simulink library "GOcontroll_Moduline_Target"  (R2023b)
settings: Solver=ode45  StartTime=0.0  StopTime=10.0  RelTol=1e-3  EnableMultiTasking=on
PreLoadFcn:
  | compile_gocontroll_mex;
libraries: $bdroot x8, canmsglib x4, simulink x2
(part 1 of 4)
settings Model: Creator=HANcoder  LastModifiedBy=maud
settings Model: ModifiedHistory=|
  | la_obwlf -- Thu Sep 01 12:12:55 2016 -- Version 0.33
  | 
  | 
  | 
  | 
  | 
  | 
  | la_obwlf -- Thu Sep 01 09:23:34 2016 -- Version 0.33
  | changed the version in the Base Sample Time block
  | 
  | 
  | 
  | la_obwlf -- Tue Aug 30 15:48:17 2016 -- Version 0.33
settings SolverCC: AlgebraicLoopSolver=TrustRegion
settings DataIOCC: LimitDataPoints=on  SaveFormat=Array  SignalLoggingSaveFormat=ModelDataLogs  ReturnWorkspaceOutputs=off
settings OptimizationCC: ExpressionDepthLimit=2147483647  LifeSpan=inf
settings DebuggingCC: UnderspecifiedInitializationDetection=Classic  MergeDetectMultiDrivingBlocksExec=none  SolverPrmCheckMsg=warning  FcnCallInpInsideContextMsg=warning  UnconnectedInputMsg=warning  UnconnectedOutputMsg=warning  UnconnectedLineMsg=warning  StateNameClashWarn=warning  SFUnexpectedBacktrackingDiag=warning  SFNoUnconditionalDefaultTransitionDiag=warning  SFExecutionAtInitializationDiag=none  ArithmeticOperatorsInVariantConditions=warning
settings HardwareCC: ProdBitPerPointer=32  ProdBitPerSizeT=32  ProdBitPerPtrDiffT=32  ProdLargestAtomicFloat=None  ProdIntDivRoundTo=Undefined  ProdEndianess=Unspecified  ProdWordSize=32  ProdHWDeviceType=32-bit Generic
settings ModelReferenceCC: EnableRefExpFcnMdlSchedulingChecks=on  PropagateSignalLabelsOutOfModel=off
settings SFSimCC: SimUseLocalCustomCode=off  CustomCodeUndefinedFunction=UseInterfaceOnly
settings RTWCC: RTWUseLocalCustomCode=off
settings CodeAppCC: StateflowObjectComments=on
settings GRTTargetCC: TargetLangStandard=C89/C90 (ANSI)  CombineOutputUpdateFcns=off  GRTInterface=on
settings ConfigComp: CovMetricSettings=dw  CovSaveCumulativeToWorkspaceVar=on  CovSaveSingleToWorkspaceVar=on  CovExternalEMLEnable=off  CovSFcnEnable=off

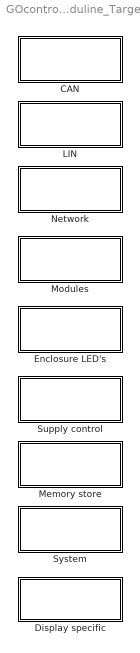
== system GOcontroll_Moduline_Target ==
  CAN : Subsystem
      mask Display: fprintf('CAN');
  Display specific : Subsystem
      mask Display: fprintf("Display specific");
  Enclosure LED's : Subsystem
      mask Display: fprintf('Enclosure LED');
  LIN : Subsystem
      mask Display: fprintf('LIN');
  Memory store : Subsystem
      mask Display: fprintf('Memory store');
  Modules : Subsystem
      mask Display: fprintf('Modules');
  Network : Subsystem
      mask Display: fprintf('Network');
  Supply control : Subsystem
      mask Display: fprintf('Supply Control');
  System : Subsystem
      mask Display: fprintf('System');

== system GOcontroll_Moduline_Target/CAN ==
  " CAN Example" : Subsystem
  CAN 2.0B : Subsystem
      mask Display: fprintf('CAN 2.0B');

== system GOcontroll_Moduline_Target/Display specific ==
  Set display brightness : M-S-Function  FunctionName=sfcn_set_brightness_display  Parameters=tsamp  mask(Set display brightness){tsamp=1}
      mask prompts: tsamp "Sample time:"
      mask help:
      | Set the brightness of a display (only works with the max25014 driver currently)
      | Keeps the original brightness untill the first non zero value is received
      mask Display:
      | fprintf("Set display brightness");
      | text(2, 6, ert_linux_target_version());

== system GOcontroll_Moduline_Target/Enclosure LED's ==
  Enclosure LED : M-S-Function  FunctionName=sfcn_gocontroll_status_led  Parameters=tsamp  mask(Enclosure LED's){tsamp=-1, led=1, color=Red}
      mask prompts: tsamp "Sample time"
      mask help:
      | The Moduline controller is equipped with 4 RGB status LED's. To control them, simply configure the mask ( LED and color) and control them using uint8 values.
      |
      | Note: Moduline IV HW >= 3.02 has duty cycle controlled LED's. The intensity can be set from 0 (0%) to 255 (100%).
      |
      | LED: Select the LED that is needs to be controlled.
      |
      | Color: Select the color the LED needs to illuminate.
      mask init:
      | colorInfoString = {'Red', 'Green', 'Blue'};
      |     colorInfoStr = colorInfoString{color};
      | 
      |     % update RTWdata to run WriteRTW again
      |     modelRTWFields = struct('led', int2str(led),'color', int2str(color));
      |     % Insert modelRTWFields in the I/O block S-Function containing the Tag starting with 'HANcoder_TARGET_'
      |     HANcoder_TARGET_DataBlock = find_system(gcb, 'RegExp', 'on', 'FollowLinks', 'on', 'LookUnderMasks', 'all', 'BlockType', 'M-S-Function');
      |     set_param(HANcoder_TARGET_DataBlock{1}, 'RTWdata', modelRTWFields);
      mask TypeOptions led: 1 | 2 | 3 | 4
      mask TypeOptions color: Red | Green | Blue
      mask Display:
      | fprintf('Status LED %d\nColor: %s',led,colorInfoStr);
      | text(2, 6, ert_linux_target_version());

== system GOcontroll_Moduline_Target/LIN ==
  LIN Master : M-S-Function  FunctionName=sfcn_lin_master  Parameters=tsamp, direction, dataLength  mask(LIN Master){id=0x01, direction=Send data, dataLength=2, check=Classic (LIN 1.3), tsamp=-1}
      mask prompts: id "Identifier"; dataLength "Data Length"; check "Checksum"; tsamp "Sample time"
      mask help:
      | Function
      | ==========
      | This block implements the LIN master functionality for communication with LIN
      | slaves. The block complies with LIN 1.3 an LIN 2.0. When sending data to a slave
      | device, this block will add the data to the LIN bus. When retrieving data from slaves, The block will wait for incoming data over LIN.
      |
      | Parameters
      | ==========
      | Identifier:
      | Selects the identifier to communicate with
      |
      | Direction:
      | Request data from a slave device or send data to a slave device
      |
      | Datalength:
      | Defines the number of bytes that need to be send to- or requested from the slave
      |
      | Checksum:
      | Select Classic for checksum based on databytes only. Enhanced for databytes and
      | ID byte
      |
      | Sample time:
      | Defines the execution interval of the block.
      |
      | Input
      | ==========
      | Port 1..8               LIN Data bytes to be send to a slave
      |
      | Output
      | ==========
      | Port 1..8               LIN Data bytes that are received from the slave
      mask init:
      | % Create resource keywords to be reserved in resource database
      | modelRTWFields = struct('id', int2str(id), 'direction', int2str(direction),'dataLength', int2str(dataLength),'check', int2str(check));
      | 
      | % Insert modelRTWFields in the I/O block S-Function containing the Tag starting with 'HANcoder_TARGET_'
      | HANcoder_TARGET_DataBlock = find_system(gcb, 'RegExp', 'on', 'FollowLinks', 'on', 'LookUnderMasks', 'all', 'BlockType', 'M-S-Function');
      | set_param(HANcoder_TARGET_DataBlock{1}, 'RTWdata', modelRTWFields);
      mask TypeOptions id: 0x01 | 0x02 | 0x03 | 0x04 | 0x05 | 0x06 | 0x07 | 0x08 | 0x09 | 0x0A | 0x0B | 0x0C | 0x0D | 0x0E | 0x0F | 0x10 | 0x11 | 0x12 | 0x13 | 0x14 | 0x15 | 0x16 | 0x17 | 0x18 | 0x19 | 0x1A | 0x1B | 0x1C | 0x1D | 0x1E | 0x1F | 0x20 | 0x21 | 0x22 | 0x23 | 0x24 | 0x25 | 0x26 | 0x27 | 0x28 | 0x29 | 0x2A | 0x2B | 0x2C | 0x2D | 0x2E | 0x2F | 0x30 | 0x31 | 0x32 | 0x33 | 0x34 | 0x35 | 0x36 | 0x37 | 0x38 | 0x39 | 0x3A | 0x3B | 0x3C (diagnostic) | 0x3D (diagnostic) | 0x3E (reserved) | 0x3F (reserved)
      mask TypeOptions direction: Request data | Send data
      mask TypeOptions dataLength: 2 | 4 | 8
      mask TypeOptions check: Classic (LIN 1.3) | Enhanced (LIN 2.0)
      mask Display:
      | fprintf('Master LIN\nmessage\nID: 0x%x',id);
      | text(2, 6, ert_linux_target_version());
      | if direction == 1
      |     port_label('output', 1, 'byte 1');
      |     port_label('output', 2, 'byte 2');
      |     if dataLength > 1
      |         port_label('output', 3, 'byte 3');
      |         port_label('output', 4, 'byte 4');
      |     end
      |     if dataLength > 2
      |         port_label('output', 5, 'byte 5');
      |         port_label('output', 6, 'byte 6');
      |         port_label('output', 7, 'byte 7');
      |         port_label('output', 8, 'byte 8');
      |     end
      | else
      |     port_label('input', 1, 'byte 1');
      |     port_label('input', 2, 'byte 2');
      |     if dataLength > 1
      |         port_label('input', 3, 'byte 3');
      |         port_label('input', 4, 'byte 4');
      |     end
      |     if dataLength > 2
      |         port_label('input', 5, 'byte 5');
      |         port_label('input', 6, 'byte 6');
      |         port_label('input', 7, 'byte 7');
      |         port_label('input', 8, 'byte 8');
      |     end
      | end

== system GOcontroll_Moduline_Target/Memory store ==
  Diagnostic to memory : Subsystem
      mask Display: fprintf('Diagnostic to memory');
  Variable to memory : Subsystem
      mask Display: fprintf('Variable to memory');

== system GOcontroll_Moduline_Target/Modules ==
  Bridge Module : Subsystem
      mask Display: fprintf('Bridge Module');
  Input Module : Subsystem
      mask Display: fprintf('Input Module');
  Output Module : Subsystem
      mask Display: fprintf('Output Module');

== system GOcontroll_Moduline_Target/Network ==
  MQTT : Subsystem  Commented=on
      mask Display: fprintf('MQTT');
  TCP : Subsystem
      mask Display: fprintf('TCP');
  UDP : Subsystem
      mask Display: fprintf('UDP');

== system GOcontroll_Moduline_Target/Supply control ==
  Controller Active : M-S-Function  FunctionName=sfcn_gocontroll_controller_active  Parameters=tsamp  mask(Controller Active){tsamp=1}
      mask prompts: tsamp "Sample time"
      mask help:
      | The GOcontroll Moduline IV is able to keep itself alive. As long the K30 power is applied (connector C pin 5-7) and the input of the Controller Active function block is high, the controller will stay on even if the K15 pins (connector C pin 2,3 or 4) are low.
      | If the controller is switched off by software, a restart is only possible when the device is activated by one of the K15 pins of connector C.
      |
      | To detect an external shutdown (K15 pins goes low), simply drag in the K15 Voltage block. This block provides the input voltage from the K15 pins
      mask Display:
      | fprintf('Controller Active');
      | text(2, 6, ert_linux_target_version());
  K15 Voltage : M-S-Function  FunctionName=sfcn_gocontroll_k15_voltage  Parameters=tsamp,k15pin  mask(Contact Voltage){ContrType=GOcontroll Moduline IV, tsamp=1, k15pin=K15-1 (Connector C pin 2)}
      mask prompts: ContrType "Controller Type"; tsamp "Sample time"; k15pin "K15 input pin"
      mask help: The K15 voltage provides the K15 voltage in mV that is applied on the K15 pins of the controller. A positive voltage on one of these pins will start-up the controller. These function blocks can be used to read out which K15 input pin triggered the startup.
      mask init:
      | %update RTWdata to run WriteRTW again
      |     modelRTWFields = struct('k15pin', int2str(k15pin));
      |     % Insert modelRTWFields in the I/O block S-Function containing the Tag starting with 'HANcoder_TARGET_'
      |     HANcoder_TARGET_DataBlock = find_system(gcb, 'RegExp', 'on', 'FollowLinks', 'on', 'LookUnderMasks', 'all', 'BlockType', 'M-S-Function');
      |     set_param(HANcoder_TARGET_DataBlock{1}, 'RTWdata', modelRTWFields);
      mask TypeOptions ContrType: GOcontroll Moduline IV | GOcontroll Moduline Mini | GOcontroll Moduline Display
      mask Callback ContrType:
      | controller = get_param(gcb, 'ContrType');
      | mask = Simulink.Mask.get(gcb);
      | adc = mask.getParameter('k15pin');
      | 
      | if(controller == "GOcontroll Moduline IV")
      |     adc.TypeOptions = {'K15-1 (Connector C pin 2)','K15-2 (Connector C pin 3)','K15-3 (Connector C pin 4)'};
      | elseif (controller == "GOcontroll Moduline Mini")
      |     adc.TypeOptions = {'K15-1 (Connector B pin 17)','K15-2 (Connector A pin 16)','K15-3 (Connector A pin 17)'};
      | elseif (controller == "GOcontroll Moduline Display")
      |     adc.TypeOptions = {'K15 (Connector A pin 9)','Sensor (6 pin Minitek pin 3)','Adapter board Sensor'};
      | end
      mask TypeOptions k15pin: K15-1 (Connector C pin 2) | K15-2 (Connector C pin 3) | K15-3 (Connector C pin 4)
      mask Display:
      | fprintf('ADC voltage\n%s',get_param(gcb, 'k15pin'));
      | text(2, 6, ert_linux_target_version());
  K30 Voltage : M-S-Function  FunctionName=sfcn_gocontroll_k30_voltage  Parameters=tsamp  mask(Supply voltage){ContrType=GOcontroll Moduline IV, tsamp=1}
      mask prompts: ContrType "Controller type"; tsamp "Sample time"
      mask help: The K30 voltage provides the power supply in mV that is applied on the K30 pins.
      mask TypeOptions ContrType: GOcontroll Moduline IV | GOcontroll Moduline Mini | GOcontroll Moduline Display
      mask Display:
      | if ContrType == 1
      |     fprintf('K30 Voltage\nConnector C pin 5-7');
      | elseif ContrType == 2
      |     fprintf('K30 Voltage\nConnector B pin 8-9');
      | elseif ContrType == 3
      |     fprintf('K30 Voltage\nConnector A pin 9');
      | end
      | text(2, 6, ert_linux_target_version());

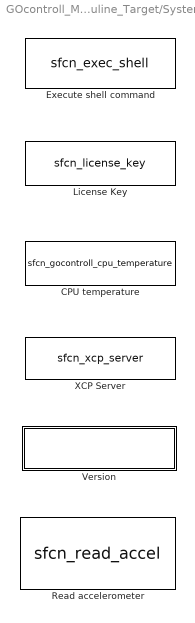
== system GOcontroll_Moduline_Target/System ==
  CPU temperature : M-S-Function  FunctionName=sfcn_gocontroll_cpu_temperature  Parameters=tsamp  mask(Get CPU temperature){tsamp=1}
      mask prompts: tsamp "Sample time"
      mask help: Block to retrieve the CPU temperature of the i.MX core
      mask Display:
      | fprintf('Get CPU temperature');
      | text(2, 6, ert_linux_target_version());
  Execute shell command : M-S-Function  FunctionName=sfcn_exec_shell  mask(Execute shell command){command='command'}
      mask help:
      | Execute a Linux Shell command when the input is true.
      |
      | Accepts a Boolean input, use a triggered subsystem to call the function only once on a state change instead of every sample.
      mask init:
      | if ~ischar(command)
      |         error('Given command is not a string');
      |     end
      | 
      |     %update RTWdata so WriteRTW gets called again
      |     modelRTWFields = struct('command', command);
      | 
      |     % Insert modelRTWFields in the I/O block S-Function containing the Tag starting with 'HANcoder_TARGET_'
      |     HANcoder_TARGET_DataBlock = find_system(gcb, 'RegExp', 'on', 'FollowLinks', 'on', 'LookUnderMasks', 'all', 'BlockType', 'M-S-Function');
      |     set_param(HANcoder_TARGET_DataBlock{1}, 'RTWdata', modelRTWFields);
      mask Display:
      | fprintf("Execute command:\n%s",command);
      | text(2, 6, ert_linux_target_version());
  License Key : M-S-Function  FunctionName=sfcn_license_key  Parameters=key,iv,license,check_file  mask(Check software license key){key=[1 2 3 4 5 6 7 8 9 10 11 12 13 14 15 16], iv='init vec', license='path/to/license', check_file='path/to/checkfile'}
      mask prompts: key "Encryption key"; iv "Initialisation vector"; license "License file"; check_file "Check file"
      mask help:
      | Function block to check the controller for a license key upon executing the software.
      |
      | example lines are literal to what should be in the field
      |
      | Encryption key:
      |
      | An array of 16, 24 or 32 bytes, for example:
      | hex2dec(["0x01", "0x23", "0x45", "0x67", "0x89", "0xAB", "0xCD", "0xEF", "0x01", "0x23", "0x45", "0x67", "0x89", "0xAB", "0xCD", "0xEF"])
      |
      | bytes can be written in any form accepted by the c compiler: 0x00/0 to 0xFf/255.
      |
      | Inititialisation vector:
      |
      | A string of characters (max 16 bytes) example:
      | '123kdgh34ndfg84'
      |
      |
      | License file:
      |
      | A string containing the path to the license file, example:
      | '/etc/simulink/license'
      |
      |
      | Check file:
      |
      | A string containing the path to the license file, example:
      | '/etc/simulink/check_file'
      |
      |
      | Method of operation:
      | This block uses the <a href="https://github.com/jhjin/OpenAES">OpenAES library</a>. It also has a tool that can be used to generate an encryption key and to encrypt a file with said key.
      |
      | This block will attempt to decrypt the "license file" with the given key and initialisation vector, it will then be compared to the "check file". If these match the program is allowed to continue.
      |
      | To make this work effectively it is essential to encrypt a file that is unique for the system and can't be easily edited. for example "/sys/class/net/eth0/address".
      |
      | An important note with using this block is that the bytes of the key are swapped and so need to be entered slightly differently in this block, for example:
      | key: byte 1 byte 2 byte 3 byte 4 byte 5 byte 6 ...
      | block: {byte 2, byte 1, byte 4, byte 3, byte 6, byte 5, ...}
      |
      | If the model terminates with the error:
      | Error: Failed to decrypt2. return code: ##
      mask init:
      | if ~(length(key) == 16 || length(key) == 24 || length(key) == 32)
      |         error('Encrypion key has an invalid length, it should be 16, 24 or 32 bytes long');
      |     end
      |     for idx = 1:length(key)
      |         if key(idx) > 255 || key(idx) < 0 || mod(key(idx),1) > 0
      |             error('Encryption key does not consist of values that match a uint8');
      |         end
      |     end
      |     if ~ischar(iv)
      |         error('Initialisation vector should be a string');
      |     end
      |     if ~ischar(license)
      |         error('Path to the license file should be a string');
      |     end
      |     if ~ischar(check_file)
      |         error('Path to the check file should be a string');
      |     end
      | 
      |     %update RTWdata here so the WriteRTW callback gets run again
      |     modelRTWFields = struct('key', mat2str(key), 'iv', iv, 'license', license, 'check_file', check_file, 'key_len', num2str(length(key)));
      | 
      |     set_param(gcb, 'RTWdata', modelRTWFields);
      mask Display:
      | fprintf('Check software license');
      | text(2, 6, ert_linux_target_version());
  Read accelerometer : M-S-Function  FunctionName=sfcn_read_accel  Parameters=tsamp  mask(Read accelerometer){sampling_frequency=12, scale=-2G/2G, tsamp=0.1}
      mask prompts: sampling_frequency "Chip sampling frequency in Hz"; scale "Sensitivity"; tsamp "Sample time"
      mask help:
      | This block reads out the accelerometer that is present on the moduline mini, other controllers will not work with this block.
      |
      | It outputs the acceleration in all 3 spatial dimensons in m/s^2.
      |
      | Positive X axis is acceleration towards the connectors in the length of the controller
      | Positive Y axis is acceleration towards the empty side of the controller, so opposite of the two m12 connectors
      | Positive Z axis is acceleration straight up if the controller was lying on its back so towards the indicator leds
      mask init:
      | switch get_param(gcb, 'scale')
      |     case '-2G/2G'
      |         scale_factor = '0.009571';
      |     case '-4G/4G'
      |         scale_factor = '0.019142';
      |     case '-8G/8G'
      |         scale_factor = '0.038285';
      |     case '-16G/16G'
      |         scale_factor = '0.076570';
      |     otherwise
      |         error('invalid sensitivity selected');
      | end
      | 
      | modelRTWFields = struct('sampling_frequency', get_param(gcb, 'sampling_frequency'), 'scale', scale_factor);
      | 
      | set_param(gcb, 'RTWdata', modelRTWFields);
      mask TypeOptions sampling_frequency: 1 | 12 | 25 | 50 | 100 | 200
      mask TypeOptions scale: -2G/2G | -4G/4G | -8G/8G | -16G/16G
      mask Display:
      | fprintf('Read accelerometer\nChip sampling frequency: %s Hz', get_param(gcb,'sampling_frequency'));
      | 
      | port_label('output', 1, 'X');
      | port_label('output', 2, 'Y');
      | port_label('output', 3, 'Z');
      | 
      | text(2, 6, ert_linux_target_version());
  Version : Subsystem  mask{major=0, feature=0, fix=1}
      mask help:
      | This block helps with keeping track of the model version.
      |
      | The values entered will be written to /usr/mem-sim/[MODEL_MAJOR,MODEL_FEATURE,MODEL_FIX].
      |
      | They are also available to use in the model with a From block, consider making them ExportedGlobal this way.
      mask init:
      | if mod(major,1) > 0
      |         error("Major must be an integer value");
      |     end
      |     if mod(feature,1) > 0
      |         error("Feature must be an integer value");
      |     end
      |     if mod(fix,1) > 0
      |         error("Fix must be an integer value");
      |     end
      mask TypeOptions major: Initialize Function/Major/Value
      mask TypeOptions feature: Initialize Function/Feature/Value
      mask TypeOptions fix: Initialize Function/Fix/Value
      mask Display:
      | fprintf('Model V%s.%s.%s', int2str(major), int2str(feature), int2str(fix));
      | text(2, 6, ert_linux_target_version());
  XCP Server : M-S-Function  Priority=999999  FunctionName=sfcn_xcp_server  mask(XCP Server){server_type=TCP}
      mask prompts: server_type "Server type"
      mask help: Having one block of this type in your model enables the XCP server to use with HANtune
      mask init:
      | %update RTWdata here so the WriteRTW callback gets run again
      |     modelRTWFields = struct('server_type', int2str(server_type));
      | 
      |     set_param(gcb, 'RTWdata', modelRTWFields);
      mask TypeOptions server_type: TCP | UDP
      mask Display:
      | fprintf('XCP Server\n%s', get_param(gcb,'server_type'));
      | text(2, 6, ert_linux_target_version());

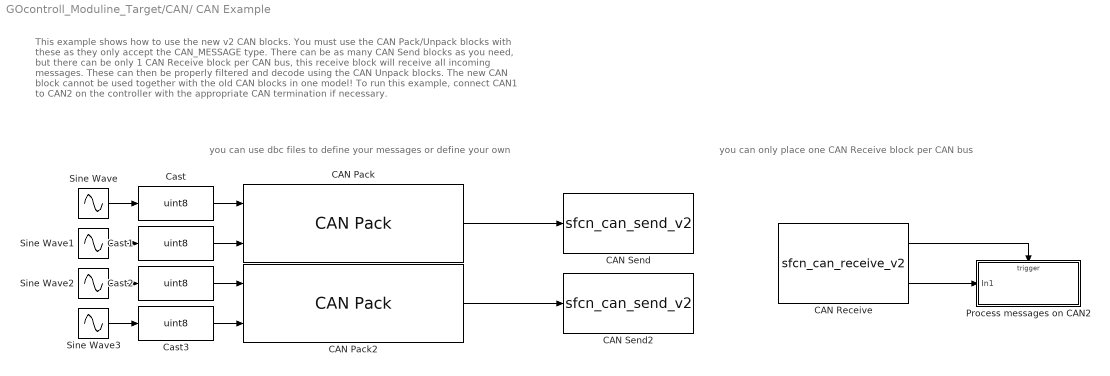
== system GOcontroll_Moduline_Target/CAN/ CAN Example ==
  note: This example shows how to use the new v2 CAN blocks.
      | You must use the CAN Pack/Unpack blocks with these as they only accept the CAN_MESSAGE type.
      | There can be as many CAN Send blocks as you need, but there can be only 1 CAN Receive block per CAN bus, this receive block will receive all incoming messages.
      | These can then be properly filtered and decode using the CAN Unpack blocks.
      | The new CAN block cannot be used together with the old CAN blocks in one model!
      |
      | To run this example, connect CAN1 to CAN2 on the controller with the appropriate CAN termination if necessary.
  note: you can use dbc files to define your messages or define your own
  note: you can only place one CAN Receive block per CAN bus
  CAN Pack : canmsglib/CAN Pack  MsgList=(none)  MsgName=CAN Msg  MsgIDType=Standard (11-bit identifier)  MsgIdentifier=10  MsgLength=2  Remote=off  ApplyMinMax=off  BusOutput=off  SignalInfo={ 'led1', '0', '8', 'LE', 'unsigned', 'Standard', '0', '1', '0', '-Inf', 'Inf'; 'led2', '8', '8', 'LE', 'unsigned', 'Standard', '0', '1', '0', '-Inf', 'Inf' }
      settings: LibrarySourceBlock=embeddedtargetslib/Host Communication/CAN Pack  DataFormat=manually specified signals
  CAN Pack2 : canmsglib/CAN Pack  MsgList=(none)  MsgName=CAN Msg  MsgIDType=Standard (11-bit identifier)  MsgIdentifier=11  MsgLength=2  Remote=off  ApplyMinMax=off  BusOutput=off  SignalInfo={ 'led3', '0', '8', 'LE', 'unsigned', 'Standard', '0', '1', '0', '-Inf', 'Inf'; 'led4', '8', '8', 'LE', 'unsigned', 'Standard', '0', '1', '0', '-Inf', 'Inf' }
      settings: LibrarySourceBlock=embeddedtargetslib/Host Communication/CAN Pack  DataFormat=manually specified signals
  CAN Receive : S-Function  AncestorBlock=GOcontroll_Moduline_Target/CAN/CAN 2.0B/CAN Receive  FunctionName=sfcn_can_receive_v2  Parameters=module_id, tsamp  SFunctionDeploymentMode=off  EnableBusSupport=off  mask(CAN Receive){ContrType=GOcontroll Moduline Mini, module_id=CAN2 - Connector A pin 24 (L) and pin 25 (H), tsamp=-1}
      mask prompts: ContrType "Controller Type"; module_id "CAN Bus"; tsamp "Sample time"
      mask help:
      | <p>Receive a messages from the CAN bus.</p>
      | <p>The output is a CAN_MESSAGE object. CAN Unpack block can be used to unpack the data from CAN_MESSAGE object.</p>
      | <p>A Function-call subsystem is triggered every time when a new message has been received.</p>
      | <p>There can be only one receive block on a given CAN bus, this receive block will receive all CAN messages on this bus. To filter them use the CAN Unpack blocks inside of a function call subsystem</p>
      mask TypeOptions ContrType: GOcontroll Moduline IV | GOcontroll Moduline Mini | GOcontroll Moduline Display
      mask Callback ContrType:
      | controller = get_param(gcb, 'ContrType');
      | mask = Simulink.Mask.get(gcb);
      | can_ifs = mask.getParameter('module_id');
      | 
      | if(controller == "GOcontroll Moduline IV")
      | can_ifs.TypeOptions = {'CAN1 - Connector C pin 14 (L) and pin 15 (H)','CAN2 - Connector C pin 20 (L) and pin 21 (H)',...
      |     'CAN3 - Connector C pin 19 (L) and pin 18 (H)','CAN4 - Connector C pin 13 (L) and pin 12 (H)'};
      | elseif (controller == "GOcontroll Moduline Mini")
      |  can_ifs.TypeOptions = {'CAN1 - Connector B pin 24 (L) and pin 25 (H)','CAN2 - Connector A pin 24 (L) and pin 25 (H)'};
      | 
      | elseif (controller == "GOcontroll Moduline Display")
      | can_ifs.TypeOptions = {'CAN1 - Connector A pin 16 (L) and pin 17 (H)','CAN2 - Connector A pin 24 (L) and pin 25 (H)'};
      | end
      mask TypeOptions module_id: CAN1 - Connector B pin 24 (L) and pin 25 (H) | CAN2 - Connector A pin 24 (L) and pin 25 (H)
      mask Display:
      | fprintf('Receive on\nCAN %x', module_id);
      | 
      | port_label('output', 1, 'function call');
      | port_label('output', 2, 'message');
      | text(2, 6, ert_linux_target_version());
  CAN Send : S-Function  AncestorBlock=GOcontroll_Moduline_Target/CAN/CAN 2.0B/CAN Send  FunctionName=sfcn_can_send_v2  Parameters=module_id, tsamp  SFunctionDeploymentMode=off  EnableBusSupport=off  mask(CAN Send){ContrType=GOcontroll Moduline Mini, module_id=CAN1, tsamp=0.01}
      mask prompts: ContrType "Controller Type"; module_id "Module"; tsamp "Sample time"
      mask help:
      | <p>Send a CAN message.</p>
      | <p>Expects a CAN_MESSAGE object as an input. Use CAN Pack to create the CAN_MESSAGE object.</p>
      mask TypeOptions ContrType: GOcontroll Moduline IV | GOcontroll Moduline Mini | GOcontroll Moduline Display
      mask Callback ContrType:
      | controller = get_param(gcb, 'ContrType');
      | mask = Simulink.Mask.get(gcb);
      | can_ifs = mask.getParameter('module_id');
      | 
      | if(controller == "GOcontroll Moduline IV")
      |     can_ifs.TypeOptions = {'CAN1 - Connector C pin 14 (L) and pin 15 (H)','CAN2 - Connector C pin 20 (L) and pin 21 (H)',...
      |         'CAN3 - Connector C pin 19 (L) and pin 18 (H)','CAN4 - Connector C pin 13 (L) and pin 12 (H)'};
      | elseif (controller == "GOcontroll Moduline Mini")
      |     can_ifs.TypeOptions = {'CAN1 - Connector B pin 24 (L) and pin 25 (H)','CAN2 - Connector A pin 24 (L) and pin 25 (H)'};
      | 
      | elseif (controller == "GOcontroll Moduline Display")
      |     can_ifs.TypeOptions = {'CAN1 - Connector A pin 16 (L) and pin 17 (H)','CAN2 - Connector A pin 24 (L) and pin 25 (H)'};
      | end
      mask TypeOptions module_id: CAN1 - Connector B pin 24 (L) and pin 25 (H) | CAN2 - Connector A pin 24 (L) and pin 25 (H)
      mask Display:
      | fprintf('Send on\nCAN%x', module_id);
      | port_label('input', 1, 'Msg');
      | 
      | text(2, 6, ert_linux_target_version());
  CAN Send2 : S-Function  AncestorBlock=GOcontroll_Moduline_Target/CAN/CAN 2.0B/CAN Send  FunctionName=sfcn_can_send_v2  Parameters=module_id, tsamp  SFunctionDeploymentMode=off  EnableBusSupport=off  mask(CAN Send){ContrType=GOcontroll Moduline Mini, module_id=CAN1, tsamp=0.01}
      mask prompts: ContrType "Controller Type"; module_id "Module"; tsamp "Sample time"
      mask help:
      | <p>Send a CAN message.</p>
      | <p>Expects a CAN_MESSAGE object as an input. Use CAN Pack to create the CAN_MESSAGE object.</p>
      mask TypeOptions ContrType: GOcontroll Moduline IV | GOcontroll Moduline Mini | GOcontroll Moduline Display
      mask Callback ContrType:
      | controller = get_param(gcb, 'ContrType');
      | mask = Simulink.Mask.get(gcb);
      | can_ifs = mask.getParameter('module_id');
      | 
      | if(controller == "GOcontroll Moduline IV")
      |     can_ifs.TypeOptions = {'CAN1 - Connector C pin 14 (L) and pin 15 (H)','CAN2 - Connector C pin 20 (L) and pin 21 (H)',...
      |         'CAN3 - Connector C pin 19 (L) and pin 18 (H)','CAN4 - Connector C pin 13 (L) and pin 12 (H)'};
      | elseif (controller == "GOcontroll Moduline Mini")
      |     can_ifs.TypeOptions = {'CAN1 - Connector B pin 24 (L) and pin 25 (H)','CAN2 - Connector A pin 24 (L) and pin 25 (H)'};
      | 
      | elseif (controller == "GOcontroll Moduline Display")
      |     can_ifs.TypeOptions = {'CAN1 - Connector A pin 16 (L) and pin 17 (H)','CAN2 - Connector A pin 24 (L) and pin 25 (H)'};
      | end
      mask TypeOptions module_id: CAN1 - Connector B pin 24 (L) and pin 25 (H) | CAN2 - Connector A pin 24 (L) and pin 25 (H)
      mask Display:
      | fprintf('Send on\nCAN%x', module_id);
      | port_label('input', 1, 'Msg');
      | 
      | text(2, 6, ert_linux_target_version());
  Cast{,1..3} (4 alike) : DataTypeConversion  OutDataTypeStr=uint8  SaturateOnIntegerOverflow=off  RndMeth=Floor
  Process messages on CAN2 : Subsystem  TreatAsAtomicUnit=on
  Sine Wave{,1..3} (4 alike) : Sin  SineType=Sample based  Amplitude=100  Bias=100  Samples=200  SampleTime=0.01
  wires:
  CAN Pack2/1 -> CAN Send2/1
  CAN Receive/2 -> Process messages on CAN2/1(In1)
  CAN Receive/1 -> Process messages on CAN2/Trigger
  Cast3/1 -> CAN Pack2/2
  Cast2/1 -> CAN Pack2/1
  Cast1/1 -> CAN Pack/2
  Sine Wave3/1 -> Cast3/1
  Sine Wave2/1 -> Cast2/1
  Sine Wave1/1 -> Cast1/1
  Sine Wave/1 -> Cast/1
  Cast/1 -> CAN Pack/1
  CAN Pack/1 -> CAN Send/1

== system GOcontroll_Moduline_Target/CAN/CAN 2.0B ==
  CAN Receive : S-Function  FunctionName=sfcn_can_receive_v2  Parameters=module_id, tsamp  SFunctionDeploymentMode=off  EnableBusSupport=off  mask(CAN Receive){ContrType=GOcontroll Moduline IV, module_id=CAN1, tsamp=-1}
      mask prompts: ContrType "Controller Type"; module_id "CAN Bus"; tsamp "Sample time"
      mask help:
      | <p>Receive a messages from the CAN bus.</p>
      | <p>The output is a CAN_MESSAGE object. CAN Unpack block can be used to unpack the data from CAN_MESSAGE object.</p>
      | <p>A Function-call subsystem is triggered every time when a new message has been received.</p>
      | <p>There can be only one receive block on a given CAN bus, this receive block will receive all CAN messages on this bus. To filter them use the CAN Unpack blocks inside of a function call subsystem</p>
      mask TypeOptions ContrType: GOcontroll Moduline IV | GOcontroll Moduline Mini | GOcontroll Moduline Display
      mask Callback ContrType:
      | controller = get_param(gcb, 'ContrType');
      | mask = Simulink.Mask.get(gcb);
      | can_ifs = mask.getParameter('module_id');
      | 
      | if(controller == "GOcontroll Moduline IV")
      | can_ifs.TypeOptions = {'CAN1 - Connector C pin 14 (L) and pin 15 (H)','CAN2 - Connector C pin 20 (L) and pin 21 (H)',...
      |     'CAN3 - Connector C pin 19 (L) and pin 18 (H)','CAN4 - Connector C pin 13 (L) and pin 12 (H)'};
      | elseif (controller == "GOcontroll Moduline Mini")
      |  can_ifs.TypeOptions = {'CAN1 - Connector B pin 24 (L) and pin 25 (H)','CAN2 - Connector A pin 24 (L) and pin 25 (H)'};
      | 
      | elseif (controller == "GOcontroll Moduline Display")
      | can_ifs.TypeOptions = {'CAN1 - Connector A pin 16 (L) and pin 17 (H)','CAN2 - Connector A pin 24 (L) and pin 25 (H)'};
      | end
      mask TypeOptions module_id: CAN1 - Connector C pin 14 (L) and pin 15 (H) | CAN2 - Connector C pin 20 (L) and pin 21 (H) | CAN3 - Connector C pin 19 (L) and pin 18 (H) | CAN4 - Connector C pin 13 (L) and pin 12 (H)
      mask Display:
      | fprintf('Receive on\nCAN %x', module_id);
      | 
      | port_label('output', 1, 'function call');
      | port_label('output', 2, 'message');
      | text(2, 6, ert_linux_target_version());
  CAN Send : S-Function  FunctionName=sfcn_can_send_v2  Parameters=module_id, tsamp  SFunctionDeploymentMode=off  EnableBusSupport=off  mask(CAN Send){ContrType=GOcontroll Moduline IV, module_id=CAN1, tsamp=0.1}
      mask prompts: ContrType "Controller Type"; module_id "CAN Bus"; tsamp "Sample time"
      mask help:
      | <p>Send a CAN message.</p>
      | <p>Expects a CAN_MESSAGE object as an input. Use CAN Pack to create the CAN_MESSAGE object.</p>
      mask TypeOptions ContrType: GOcontroll Moduline IV | GOcontroll Moduline Mini | GOcontroll Moduline Display
      mask Callback ContrType:
      | controller = get_param(gcb, 'ContrType');
      | mask = Simulink.Mask.get(gcb);
      | can_ifs = mask.getParameter('module_id');
      | 
      | if(controller == "GOcontroll Moduline IV")
      |     can_ifs.TypeOptions = {'CAN1 - Connector C pin 14 (L) and pin 15 (H)','CAN2 - Connector C pin 20 (L) and pin 21 (H)',...
      |         'CAN3 - Connector C pin 19 (L) and pin 18 (H)','CAN4 - Connector C pin 13 (L) and pin 12 (H)'};
      | elseif (controller == "GOcontroll Moduline Mini")
      |     can_ifs.TypeOptions = {'CAN1 - Connector B pin 24 (L) and pin 25 (H)','CAN2 - Connector A pin 24 (L) and pin 25 (H)'};
      | 
      | elseif (controller == "GOcontroll Moduline Display")
      |     can_ifs.TypeOptions = {'CAN1 - Connector A pin 16 (L) and pin 17 (H)','CAN2 - Connector A pin 24 (L) and pin 25 (H)'};
      | end
      mask TypeOptions module_id: CAN1 - Connector C pin 14 (L) and pin 15 (H) | CAN2 - Connector C pin 20 (L) and pin 21 (H) | CAN3 - Connector C pin 19 (L) and pin 18 (H) | CAN4 - Connector C pin 13 (L) and pin 12 (H)
      mask Display:
      | fprintf('Send on\nCAN%x', module_id);
      | port_label('input', 1, 'Msg');
      | 
      | text(2, 6, ert_linux_target_version());
  CAN receive1 : M-S-Function  FunctionName=sfcn_can_receive  Parameters=tsamp,canBus,outputNumber,dataType, byteOrder  mask(CAN receive (Legacy)){ContrType=GOcontroll Moduline IV, canBus=CAN1 - Connector C pin 14 (L) and pin 15 (H), outputNumber=1, dataType=uint8, byteOrder=on, tsamp=-1}
      mask prompts: ContrType "Controller Type"; canBus "CAN channel"; outputNumber "Output ports"; dataType "Output datatype"; byteOrder "Byte order: Checked = MSB first, unchecked = LSB first."; tsamp "Sample time"
      mask help:
      | !! Legacy block, use the CAN receive instead of CAN receive1 in future projects !!
      | !! These will not work together, either use the legacy blocks or the new ones !!
      |
      | Function
      | ==========
      | Receive the newest message from the specified CAN channel.
      |
      | Parameters
      | ==========
      | Controller Type          The controller type, only changes the available CAN channels and puts the correct pinout for that type
      | CAN channel:             The CAN channel to send the message on.
      | Output ports:             The amount of output ports
      | Output datatype:       The datatype of the output ports
      | Byte order:                 Select MSB or LSB first
      | Sample time:              -1 or divisible by base sample time [seconds]
      |
      | Input
      | ==========
      | Port 1:                       CAN ID(uint32) in hexadecimal ie: hex2dec('0a')
      |
      | Output
      | ==========
      | Port 1:                       Checks for new message(int8)
      | Port 2..9                     Message data
      mask init:
      | % calculate the data length (targe specific)
      | dataLength = 0;
      | switch(dataType)
      |     case {1,2,7}
      |         % data length of 1 byte
      |         dataLength = outputNumber * 1;
      |     case {3,4}
      |         % data length of 2 bytes
      |         dataLength = outputNumber * 2;
      |     case {5,6}
      |         % data length of 4 bytes
      |         dataLength = outputNumber * 4;
      | end
      | 
      | % check if number of outputs, combined with the data type, is exceeding the
      | % maximum data length
      | if (dataLength < 1)
      |     error ('The CAN message has a minimum of 1 byte');
      | elseif (dataLength > 8)
      |     error('The CAN message supports only up to 8 data bytes');
      | end
      | 
      | % Create resource keywords to be reserved in resource database
      | modelRTWFields = struct('canBus', int2str(canBus-1),...
      |     'outputNumber', int2str(outputNumber), 'dataType', int2str(dataType), 'byteOrder', int2str(byteOrder),...
      |     'dataLength', int2str(dataLength));
      | 
      | set_param(gcb, 'RTWdata', modelRTWFields);
      mask TypeOptions ContrType: GOcontroll Moduline IV | GOcontroll Moduline Mini | GOcontroll Moduline Display
      mask Callback ContrType:
      | controller = get_param(gcb, 'ContrType');
      | mask = Simulink.Mask.get(gcb);
      | can_ifs = mask.getParameter('canBus');
      | 
      | if(controller == "GOcontroll Moduline IV")
      |     can_ifs.TypeOptions = {'CAN1 - Connector C pin 14 (L) and pin 15 (H)','CAN2 - Connector C pin 20 (L) and pin 21 (H)',...
      |         'CAN3 - Connector C pin 19 (L) and pin 18 (H)','CAN4 - Connector C pin 13 (L) and pin 12 (H)'};
      | elseif (controller == "GOcontroll Moduline Mini")
      |     can_ifs.TypeOptions = {'CAN1 - Connector B pin 24 (L) and pin 25 (H)','CAN2 - Connector A pin 24 (L) and pin 25 (H)'};
      | 
      | elseif (controller == "GOcontroll Moduline Display")
      |     can_ifs.TypeOptions = {'CAN1 - Connector A pin 16 (L) and pin 17 (H)','CAN2 - Connector A pin 24 (L) and pin 25 (H)'};
      | end
      mask TypeOptions canBus: CAN1 - Connector C pin 14 (L) and pin 15 (H) | CAN2 - Connector C pin 20 (L) and pin 21 (H) | CAN3 - Connector C pin 19 (L) and pin 18 (H) | CAN4 - Connector C pin 13 (L) and pin 12 (H)
      mask TypeOptions dataType: int8 | uint8 | int16 | uint16 | int32 | uint32 | boolean
      mask Display:
      | fprintf('Receive on\nCAN %x', canBus);
      | port_label('output', 1, 'new')
      | port_label('input', 1, 'ID');
      | text(2, 6, ert_linux_target_version());
  CAN send1 : M-S-Function  FunctionName=sfcn_can_send  Parameters=tsamp, canBus, frameType, inputNumber,RTR  mask(CAN send (Legacy)){ContrType=GOcontroll Moduline IV, canBus=CAN1 - Connector C pin 14 (L) and pin 15 (H), frameType=Standard (11 bit), inputNumber=1, RTR=off, tsamp=-1}
      mask prompts: ContrType "Controller Type"; canBus "CAN channel"; frameType "Identifier type"; inputNumber "Input ports"; RTR "Remote Transmission Request"; tsamp "Sample time"
      mask help:
      | !! Legacy block, use the CAN send instead of CAN send1 in future projects !!
      | !! These will not work together, either use the legacy blocks or the new ones !!
      |
      |
      | Function
      | ==========
      | Send a message on the CAN channel.
      |
      | Parameters
      | ==========
      | Controller Type        The controller type, only changes the available CAN channels and puts the correct pinout for that type
      | CAN channel:           The CAN channel to send the message on.
      | Identifier type:         normal or extended ID's
      | Input ports:              The amount of input ports
      | Sample time:            -1 or divisible by base sample time [seconds]
      |
      | Input
      | ==========
      | Port 1:                   CAN ID(uint32) in hexadecimal ie: hex2dec('0a')
      | Port 2..9                CAN message data (uint8)
      mask init:
      | % check if number of inputs, combined with the data type, is exceeding the
      | % maximum data length
      | if (inputNumber > 8)
      |     error('The CAN message supports only up to 8 data bytes');
      | elseif (inputNumber < 0)
      | 	error('The CAN message cant have a negative number of bytes');
      | end
      | 
      | % Create resource keywords to be reserved in resource database
      | modelRTWFields = struct('canBus', int2str(canBus-1), 'frameType', int2str(frameType),...
      |     'inputNumber', int2str(inputNumber), 'dataLength', int2str(inputNumber), 'RTR', int2str(RTR));
      | 
      | set_param(gcb, 'RTWdata', modelRTWFields);
      mask TypeOptions ContrType: GOcontroll Moduline IV | GOcontroll Moduline Mini | GOcontroll Moduline Display
      mask Callback ContrType:
      | controller = get_param(gcb, 'ContrType');
      | mask = Simulink.Mask.get(gcb);
      | can_ifs = mask.getParameter('canBus');
      | 
      | if(controller == "GOcontroll Moduline IV")
      |     can_ifs.TypeOptions = {'CAN1 - Connector C pin 14 (L) and pin 15 (H)','CAN2 - Connector C pin 20 (L) and pin 21 (H)',...
      |         'CAN3 - Connector C pin 19 (L) and pin 18 (H)','CAN4 - Connector C pin 13 (L) and pin 12 (H)'};
      | elseif (controller == "GOcontroll Moduline Mini")
      |     can_ifs.TypeOptions = {'CAN1 - Connector B pin 24 (L) and pin 25 (H)','CAN2 - Connector A pin 24 (L) and pin 25 (H)'};
      | 
      | elseif (controller == "GOcontroll Moduline Display")
      |     can_ifs.TypeOptions = {'CAN1 - Connector A pin 16 (L) and pin 17 (H)','CAN2 - Connector A pin 24 (L) and pin 25 (H)'};
      | end
      mask TypeOptions canBus: CAN1 - Connector C pin 14 (L) and pin 15 (H) | CAN2 - Connector C pin 20 (L) and pin 21 (H) | CAN3 - Connector C pin 19 (L) and pin 18 (H) | CAN4 - Connector C pin 13 (L) and pin 12 (H)
      mask TypeOptions frameType: Standard (11 bit) | Extended (29 bit)
      mask Display:
      | fprintf('Send on\nCAN%x', canBus);
      | port_label('input', 1, 'ID');
      | if RTR
      |     fprintf('\n\n\n\nRTR');
      | end
      | text(2, 6, ert_linux_target_version());

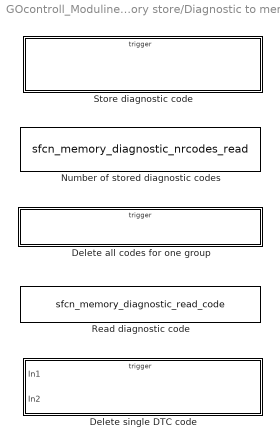
== system GOcontroll_Moduline_Target/Memory store/Diagnostic to memory ==
  Delete all codes for one group : Subsystem  mask(Delete diagnostic codes from memory){TriggerType=rising}
      mask prompts: TriggerType "Simulink:blkprm_prompts:TrigPortTrigType"
      mask help:
      | This function block deletes stored codes under the specified diagnostic code type.
      |
      | Diagnostic code type:
      | The type defines the severity of the diagnostic code categorie that is deleted.
      mask TypeOptions TriggerType: Trigger/TriggerType
      mask DialogControl TriggerType Prompt: Trigger type:
      mask Display:
      | fprintf('Delete all DTCs');
      | text(2, 6, ert_linux_target_version());
  Delete single DTC code : Subsystem  TreatAsAtomicUnit=on  mask(Store diagnostic code to memory){TriggerType=rising}
      mask prompts: TriggerType "Simulink:blkprm_prompts:TrigPortTrigType"
      mask help:
      | This function block stores a diagnostic code to memory.
      |
      | Diagnostic code type:
      | The type defines the severity of the diagnostic code.
      mask init:
      | % array with module slot infos
      mask TypeOptions TriggerType: Trigger/TriggerType
      mask DialogControl TriggerType Prompt: Trigger type:
      mask Display:
      | fprintf('Delete single DTC from memory');
      | port_label('input', 1, 'SPN');
      | port_label('input', 2, 'FMI');
      | text(2, 6, ert_linux_target_version());
  Number of stored diagnostic codes : M-S-Function  FunctionName=sfcn_memory_diagnostic_nrcodes_read  Parameters=tsamp  mask(Read number of stored codes){tsamp=0.5}
      mask prompts: tsamp "Sample time"
      mask help:
      | This function block reads the number of stored codes under the specified diagnostic code type.
      |
      | Sample time:
      | Execution period for the function block.
      | You might want to put this block in a triggered subsystem or a function call subsystem
      |
      | Diagnostic code type:
      | The type defines the severity of the diagnostic code categorie that is read.
      mask init:
      | % Insert modelRTWFields in the I/O block S-Function containing the Tag starting with 'HANcoder_TARGET_'
      | HANcoder_TARGET_DataBlock = find_system(gcb, 'RegExp', 'on', 'FollowLinks', 'on', 'LookUnderMasks', 'all', 'BlockType', 'M-S-Function');
      | %set_param(HANcoder_TARGET_DataBlock{1}, 'RTWdata', modelRTWFields);
      mask Display:
      | fprintf('Get number of stored DTCs');
      | text(2, 6, ert_linux_target_version());
  Read diagnostic code : M-S-Function  FunctionName=sfcn_memory_diagnostic_read_code  Parameters=tsamp  mask(Read a diagnostic code from memory){tsamp=0.5}
      mask prompts: tsamp "Sample time"
      mask help:
      | This function block reads a stored diagnostic code from memory. The code that is read from memory is specified by the index numper on input port 1. The stored code goes out of the functionblock as a uint32 value.
      |
      | Sample time:
      | Execution period for the function block.
      |
      | It might be a good idea to use this block in a triggered subsystem or a function call subsystem
      mask Display:
      | fprintf('Read DTC from index');
      | port_label('input', 1, 'Index');
      | port_label('output', 1, 'Code');
      | text(2, 6, ert_linux_target_version());
  Store diagnostic code : Subsystem  TreatAsAtomicUnit=on  mask(Store diagnostic code to memory){spn=1234, fmi=(0) Data valid but above normal operational range, most severe level (3)}
      mask prompts: spn "SPN number"; fmi "Failer Mode Indicator"
      mask help:
      | This function block stores a diagnostic code to memory.
      |
      | Diagnostic code type:
      | The type defines the severity of the diagnostic code.
      mask TypeOptions spn: Store DTC code/spn
      mask TypeOptions fmi: Store DTC code/fmi
      mask Display:
      | fprintf('Store DTC to memory\n SPN: %d\n FMI: %d',spn, fmi);
      | text(2, 6, ert_linux_target_version());

== system GOcontroll_Moduline_Target/Memory store/Variable to memory ==
  Memory read : M-S-Function  FunctionName=sfcn_memory_emulation_read  Parameters=tsamp  mask(Read value from memory){memRead=Read once during startup, memType=Persistant Memory (eMMC), tsamp=1, key=key, init=0}
      mask prompts: memRead "Memory read"; memType "Memory type"; tsamp "Sample time"; init "Initialization value"
      mask help: This function block reads a value from memory by the specified key. To store a value to memory, use the store to memory function block.
      mask init:
      | % update RTWdata so WriteRTW gets called when building the model
      |     modelRTWFields = 	struct( 'memRead', int2str(memRead), 'memType', int2str(memType),'key', key, 'init', int2str(init));
      |     
      |     % Insert modelRTWFields in the I/O block S-Function containing the Tag starting with 'HANcoder_TARGET_'
      |     HANcoder_TARGET_DataBlock = find_system(gcb, 'RegExp', 'on', 'FollowLinks', 'on', 'LookUnderMasks', 'all', 'BlockType', 'M-S-Function');
      |     set_param(HANcoder_TARGET_DataBlock{1}, 'RTWdata', modelRTWFields);
      mask TypeOptions memRead: Read once during startup | Read periodic based on sample time
      mask TypeOptions memType: Persistant Memory (eMMC) | Non-persistant Memory (RAM) | Configuration (eMMC)
      mask Display:
      | fprintf('Read from memory\nKey: %s',key);
      | text(2, 6, ert_linux_target_version());
  Memory write : M-S-Function  FunctionName=sfcn_memory_emulation_write  Parameters=tsamp  mask(Store data to memory){memType=Persistant Memory (eMMC), tsamp=1, key=key}
      mask prompts: memType "Memory type"; tsamp "Sample time"
      mask help: This function block stores a value to the memory with a specified key. To get the stored value from memory, use the read from memory function block and retrieve the value by key
      mask init:
      | %update RTWdata so WriteRTW param gets called again
      |     modelRTWFields = struct('key', key,  'memType', int2str(memType));
      | 
      |     % Insert modelRTWFields in the I/O block S-Function containing the Tag starting with 'HANcoder_TARGET_'
      |     HANcoder_TARGET_DataBlock = find_system(gcb, 'RegExp', 'on', 'FollowLinks', 'on', 'LookUnderMasks', 'all', 'BlockType', 'M-S-Function');
      |     set_param(HANcoder_TARGET_DataBlock{1}, 'RTWdata', modelRTWFields);
      mask TypeOptions memType: Persistant Memory (eMMC) | Non-persistant Memory (RAM)
      mask Display:
      | fprintf('Store in memory\nKey: %s',key);
      | text(2, 6, ert_linux_target_version());
